simulink model "fig2_1_simulink"  (R2021b)
settings: Solver=ode45  StartTime=0.0  StopTime=1.7  RelTol=1e-3  EnableMultiTasking=on
model workspace (MAT data in the model file):
  X0 = 0
settings Model: Creator=One Informatic  LastModifiedBy=One Informatic
settings DataIOCC: LimitDataPoints=on  SaveFormat=Array  SignalLoggingSaveFormat=ModelDataLogs  ReturnWorkspaceOutputs=off  SignalLoggingName=sigsOut
settings DebuggingCC: SaveWithParameterizedLinksMsg=none  UnderspecifiedInitializationDetection=Classic  MergeDetectMultiDrivingBlocksExec=none  SignalResolutionControl=TryResolveAllWithWarning  MultiTaskDSMMsg=warning  MultiTaskCondExecSysMsg=none
settings HardwareCC: ProdBitPerPointer=32  ProdBitPerSizeT=32  ProdBitPerPtrDiffT=32  ProdLargestAtomicFloat=None  ProdIntDivRoundTo=Undefined  ProdEndianess=Unspecified  ProdWordSize=32  ProdHWDeviceType=32-bit Generic  TargetUnknown=on
settings ModelReferenceCC: PropagateSignalLabelsOutOfModel=off
settings GRTTargetCC: CombineOutputUpdateFcns=off  GRTInterface=on
settings ConfigComp: CovMetricSettings=dw  CovSaveCumulativeToWorkspaceVar=on  CovSaveSingleToWorkspaceVar=on

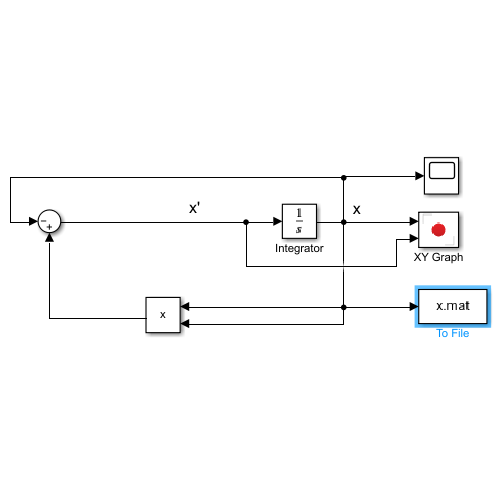
[thumbnail: Simulink's stored preview of the top-level diagram]
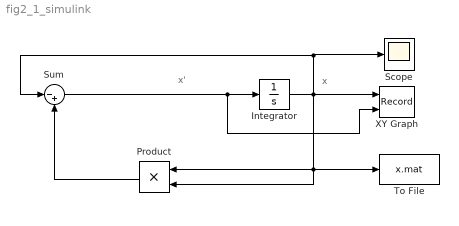
== system fig2_1_simulink ==
  note: x'
  note: x
  Integrator : Integrator  InitialCondition=1.2
  Product : Product
  Scope : Scope
  Sum : Sum  Inputs=|-+
  To File : ToFile  Filename=x.mat  MatrixName=x  SampleTime=0.001
  XY Graph : Record  FileSettingsInternal="{\"entries\":[{\"content\":{\"excelSettings\":{\"content\":{},\"type\":\"Streamout.ExcelSettings\"}},\"type\":\"Streamout.FileSettingStorage\",\"uuid\":\"c7d7ec70-e5b2-4626-a0cd-61a9e9ace36f\"}],\"packageUris\":[\"http://schema.mathworks.com/mf0/streamout_blocks/R2020a\"],\"version\":\"1.0\"}"  Layout=[1 1]  SignalsInternal="{\"entries\":[{\"content\":{\"signals\":[{\"content\":{\"blockPath\":[\"fig2_1_simulink/XY Graph\"],\"channel\":[],\"dimensions\":[1],\"domain\":\"fig2_1_simulink/XY Graph\",\"lineColor\":\"#a2142f\",\"plots\":[1],\"port\":1,\"sid\":[\"\"],\"signalID\":299,\"signalName\":\"Integrator\"},\"type\":\"RecordBlkView.Signal\",\"uuid\":\"2ec07001-44e3-40f7-9b6b-57d81be30820\"},{\"content\":{\"blockPath\":[\"fig2_1_simulink/XY Graph\"],\"channel\":[],\"dimensions\":[1],\"domain\":\"fig2_1_simulink/XY Graph\",\"lineColor\":\"#139fff\",\"plots\":[1],\"port\":2,\"sid\":[\"\"],\"signalID\":303,\"signalName\":\"Sum\"},\"type\":\"RecordBlkView.Signal\",\"uuid\":\"c64fd694-fc12-4e5c-9478-cb3b1a2be2f9\"}]},\"type\":\"RecordBlkView.InputSignals\",\"uuid\":\"959e94c7-bc41-493a-9980-313c6f66fdb4\"}],\"packageUris\":[\"http://schema.mathworks.com/mf0/streamout_blocks/R2020a\"],\"version\":\"1.0\"}"  VisualizationBindings="{\"xyplotplugin\":{\"info\":[{\"series\":[{\"bindingParametersList\":[{\"parameter\":\"X-Axis\",\"signalID\":299,\"signalName\":\"Integrator\"},{\"parameter\":\"Y-Axis\",\"signalID\":303,\"signalName\":\"Sum\"}],\"seriesID\":16801}],\"subplotID\":1}]}}"  CompatibilityTag=XY
  wires:
  Product/1 -> Sum/2
  Sum/1 -> XY Graph/2, Integrator/1
  Integrator/1 -> Scope/1, Sum/1, To File/1, Product/2, Product/1, XY Graph/1
